simulink model "inverted_pendulum"  (R2021a)
settings: Solver=VariableStepAuto  StartTime=0.0  StopTime=5  FixedStep=0.001  MaxStep=0.0001  RelTol=1e-3
values from neighbouring files (symbols this model uses):
  A = [0          1       0       0 ... (first row only)    [Data.m]
  B = [0 0 0 1/La]'    [Data.m]
  beta = g*(mp*L1 + mw * L2)    (= 0.64746)    [Data.m]    (also in uncertainty.m = g*(mp*L1 + mw * L2))
  bm = 0.018    [Data.m]    (also in uncertainty.m = ureal('bm', 0.018, 'percent', 20))
  bp = 0.038    [Data.m]    (also in uncertainty.m = ureal('bp', 0.038, 'percent', 100))
  C = [1 0 0 0]    [Data.m]
  fs_IMU = 1000    [Data.m]
  g = 9.81    [Data.m]    (also in uncertainty.m)
  ideal_acc_height = 0    [Data.m]
  J1 = Jw + Jp_O    (= 0.0170488)    [Data.m]    (also in uncertainty.m = Jw + Jp_O)
  Jw = J_motor + J_wheel    (= 0.0042488)    [Data.m]    (also in uncertainty.m = J_motor + J_wheel)
  Ke = 1.66e-2    (= 0.0166)    [Data.m]    (also in gear_test.m = gear*Kt; uncertainty.m = ureal('Ke', 1.66e-2, 'percent', 20))
  Ksw = 0.035    [Data.m]    (also in Ksw_test.m = Ksw_v(i))
  Kt = 1    [Data.m]    (also in gear_test.m = gear*0.876; uncertainty.m = ureal('Kt', 1, 'percent', 20))
  L = L_t'    [Data.m]
  La = 3.2e-3    (= 0.0032)    [Data.m]    (also in uncertainty.m = ureal('La', 3.2e-3, 'percent', 20))
  Ra = 40.8    [Data.m]    (also in uncertainty.m = ureal('Ra', 40.8, 'percent', 20))
  real_acc_height = 0.02    [Data.m]
  V_nom = 24    [Data.m]    (also in uncertainty.m)
  wd_IMU = 30000*2*pi    (= 188495.559215)    [Data.m]
  wn = sqrt(mp*g*L2/Jp_O)    [Data.m]
  x0 = [0.3 0 0 0]    [Data.m]
  x0_sw = [pi 0 0 0]    [Data.m]    (also in phase_space.m = [-pi 0 0 0])
undefined symbols (not defined in the file or in its folder): acc_bias, gyro_bias, K
libraries: spsFirstOrderFilterLib x18, simulink x9, dspsigops x2
(part 2 of 2)

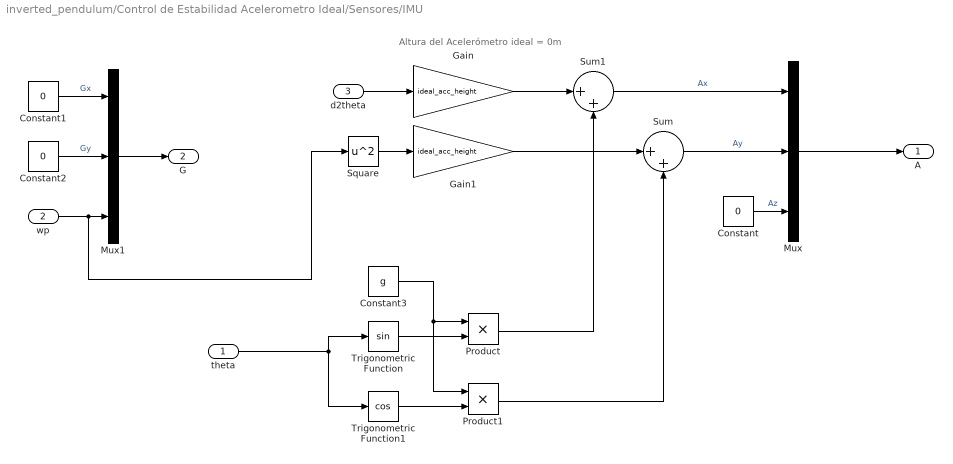
== system inverted_pendulum/Control de Estabilidad Acelerometro Ideal/Sensores/IMU ==
  note: Altura del Acelerómetro ideal = 0m
  theta : Inport
  wp : Inport  Port=2
  d2theta : Inport  Port=3
  Constant : Constant  Value=0
  Constant1 : Constant  Value=0
  Constant2 : Constant  Value=0
  Constant3 : Constant  Value=g
  Gain : Gain  Gain=ideal_acc_height
  Gain1 : Gain  Gain=ideal_acc_height
  Mux : Mux  Inputs=3
  Mux1 : Mux  Inputs=3
  Product : Product
  Product1 : Product
  Square : Math  Operator=square  SaturateOnIntegerOverflow=on
  Sum : Sum  Inputs=|++
  Sum1 : Sum  Inputs=|++
  Trigonometric Function : Trigonometry
  Trigonometric Function1 : Trigonometry  Operator=cos
  A : Outport
  G : Outport  Port=2
  wires:
  Mux/1 -> A/1
  Mux1/1 -> G/1
  Sum/1 -> Mux/2  "Ay"
  Constant/1 -> Mux/3  "Az"
  Sum1/1 -> Mux/1  "Ax"
  Constant2/1 -> Mux1/2  "Gy"
  Constant1/1 -> Mux1/1  "Gx"
  wp/1 -> Square/1, Mux1/3
  Trigonometric Function/1 -> Product/2
  Trigonometric Function1/1 -> Product1/2
  Constant3/1 -> Product1/1, Product/1
  Product1/1 -> Sum/2
  Product/1 -> Sum1/2
  Gain1/1 -> Sum/1
  theta/1 -> Trigonometric Function1/1, Trigonometric Function/1
  Gain/1 -> Sum1/1
  d2theta/1 -> Gain/1
  Square/1 -> Gain1/1

== system inverted_pendulum/Control de Estabilidad Acelerometro Real/Péndulo invertido NL/Motor CC + Rueda ==
  note: Rueda
  note: Motor CC
  V : Inport
  Gain : Gain  Gain=1/Jw
  Gain1 : Gain  Gain=bm
  Gain2 : Gain  Gain=Kt
  Gain3 : Gain  Gain=1/La
  Gain4 : Gain  Gain=Ra
  Gain5 : Gain  Gain=Ke
  Integrator ia : Integrator  InitialCondition=x0(4)
  Integrator wm : Integrator  InitialCondition=x0(3)
  Sum : Sum  Inputs=|+-
  Sum1 : Sum  Inputs=|+--
  wm : Outport
  ia : Outport  Port=2
  wires:
  Sum/1 -> Gain/1
  Gain/1 -> Integrator wm/1  "d2phi"
  Integrator wm/1 -> wm/1, Gain1/1, Gain5/1  "wm"
  Gain1/1 -> Sum/2
  Gain2/1 -> Sum/1
  Integrator ia/1 -> ia/1, Gain4/1, Gain2/1  "ia"
  Gain3/1 -> Integrator ia/1  "di/dt"
  Sum1/1 -> Gain3/1
  Gain4/1 -> Sum1/3
  V/1 -> Sum1/1  "V"
  Gain5/1 -> Sum1/2

== system inverted_pendulum/Control de Estabilidad Acelerometro Real/Péndulo invertido NL/Péndulo invertido ==
  note: Péndulo
  note: Fricción del motor
  note: Torque del motor
  wm : Inport
  ia : Inport  Port=2
  Gain : Gain  Gain=1/J1
  Gain1 : Gain  Gain=beta
  Gain2 : Gain  Gain=Kt
  Gain3 : Gain  Gain=bp
  Gain4 : Gain  Gain=bm
  Integrator Theta : Integrator  InitialCondition=x0(1)  WrappedStateUpperValue=2*pi  WrappedStateLowerValue=0
  Integrator wp : Integrator  InitialCondition=x0(2)
  Sum : Sum  Inputs=+-+-
  Trigonometric Function1 : Trigonometry
  theta : Outport
  wp : Outport  Port=2
  d2theta : Outport  Port=3
  wires:
  Trigonometric Function1/1 -> Gain1/1
  Gain/1 -> d2theta/1, Integrator wp/1  "d2theta"
  Sum/1 -> Gain/1
  Integrator Theta/1 -> Trigonometric Function1/1, theta/1  "theta"
  Integrator wp/1 -> wp/1, Gain3/1, Integrator Theta/1  "wp"
  Gain3/1 -> Sum/4
  Gain1/1 -> Sum/3
  ia/1 -> Gain2/1
  Gain2/1 -> Sum/2
  wm/1 -> Gain4/1
  Gain4/1 -> Sum/1

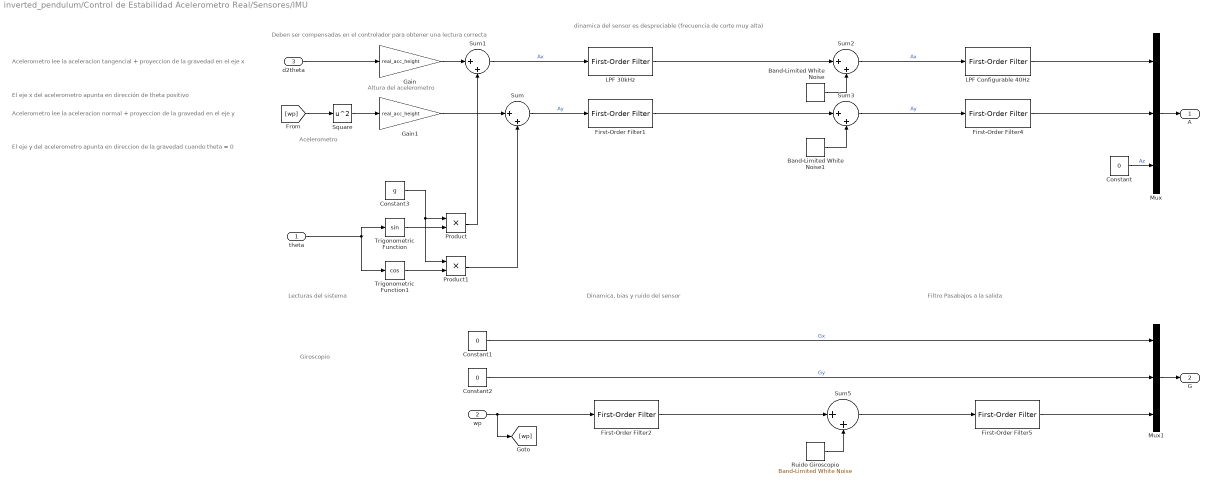
== system inverted_pendulum/Control de Estabilidad Acelerometro Real/Sensores/IMU ==
  note: dinamica del sensor es despreciable (frecuencia de corte muy alta)
  note: Dinamica, bias y ruido del sensor
  note: Lecturas del sistema
  note: Acelerometro
  note: Deben ser compensadas en el controlador para obtener una lectura correcta
  note: Acelerometro lee la aceleracion tangencial + proyeccion de la gravedad en el eje x
  note: Altura del acelerometro
  note: El eje y del acelerometro apunta en direccion de la gravedad cuando theta = 0
  note: El eje x del acelerometro apunta en dirección de theta positivo
  note: Acelerometro lee la aceleracion normal + proyeccion de la gravedad en el eje y
  note: Giroscopio
  note: Filtro Pasabajos a la salida
  theta : Inport
  wp : Inport  Port=2
  d2theta : Inport  Port=3
  Band-Limited White Noise : simulink/Sources/Band-Limited White Noise  Cov=acc_noise_power  Ts=1/fs_IMU  seed=[23341]
  Band-Limited White Noise1 : simulink/Sources/Band-Limited White Noise  Cov=acc_noise_power  Ts=1/fs_IMU  seed=[23341]
  Constant : Constant  Value=0
  Constant1 : Constant  Value=0
  Constant2 : Constant  Value=0
  Constant3 : Constant  Value=g
  First-Order Filter{1..2,4..5} (4 alike) : spsFirstOrderFilterLib/First-Order Filter  FilterType=Lowpass  Tc=2*pi/wd_IMU  Ts=0  Initialize=on  Vac_Init=[0, 0, 60]  Vdc_Init=0  PlotResponse=off  FreqRange="[0,  200,  1]"
  Gain : Gain  Gain=real_acc_height
  Gain1 : Gain  Gain=real_acc_height
  LPF 30kHz : spsFirstOrderFilterLib/First-Order Filter  FilterType=Lowpass  Tc=2*pi/wd_IMU  Ts=0  Initialize=on  Vac_Init=[0, 0, 60]  Vdc_Init=0  PlotResponse=off  FreqRange="[0,  200,  1]"
  LPF Configurable 40Hz : spsFirstOrderFilterLib/First-Order Filter  FilterType=Lowpass  Tc=2*pi/wd_IMU  Ts=0  Initialize=on  Vac_Init=[0, 0, 60]  Vdc_Init=0  PlotResponse=off  FreqRange="[0,  200,  1]"
  Mux : Mux  Inputs=3
  Mux1 : Mux  Inputs=3
  Product : Product
  Product1 : Product
  Ruido Giroscopio : simulink/Sources/Band-Limited White Noise  Cov=gyro_noise_power  Ts=1/fs_IMU  seed=[23341]
  Square : Math  Operator=square  SaturateOnIntegerOverflow=on
  Sum{,1..3,5} (5 alike) : Sum  Inputs=|++
  Trigonometric Function : Trigonometry
  Trigonometric Function1 : Trigonometry  Operator=cos
  A : Outport
  G : Outport  Port=2
  wires:
  Constant2/1 -> Mux1/2  "Gy"
  Constant1/1 -> Mux1/1  "Gx"
  Trigonometric Function/1 -> Product/2
  Trigonometric Function1/1 -> Product1/2
  Constant3/1 -> Product1/1, Product/1
  Product1/1 -> Sum/2
  Product/1 -> Sum1/2
  Gain1/1 -> Sum/1
  theta/1 -> Trigonometric Function1/1, Trigonometric Function/1
  Gain/1 -> Sum1/1
  d2theta/1 -> Gain/1
  Square/1 -> Gain1/1
  Constant/1 -> Mux/3  "Az"
  Sum1/1 -> LPF 30kHz/1  "Ax"
  Band-Limited White Noise/1 -> Sum2/2
  Band-Limited White Noise1/1 -> Sum3/2
  Ruido Giroscopio/1 -> Sum5/2
  First-Order Filter1/1 -> Sum3/1
  First-Order Filter2/1 -> Sum5/1
  wp/1 -> First-Order Filter2/1, [wp]
  Mux/1 -> A/1
  Mux1/1 -> G/1
  Sum5/1 -> First-Order Filter5/1
  Sum2/1 -> LPF Configurable 40Hz/1  "Ax"
  Sum3/1 -> First-Order Filter4/1  "Ay"
  [wp] -> Square/1
  Sum/1 -> First-Order Filter1/1  "Ay"
  LPF 30kHz/1 -> Sum2/1
  First-Order Filter4/1 -> Mux/2
  LPF Configurable 40Hz/1 -> Mux/1
  First-Order Filter5/1 -> Mux1/3

== system inverted_pendulum/Control de Estabilidad Sensores ideales/Péndulo invertido NL/Motor CC + Rueda ==
  note: Rueda
  note: Motor CC
  V : Inport
  Gain : Gain  Gain=1/Jw
  Gain1 : Gain  Gain=bm
  Gain2 : Gain  Gain=Kt
  Gain3 : Gain  Gain=1/La
  Gain4 : Gain  Gain=Ra
  Gain5 : Gain  Gain=Ke
  Integrator ia : Integrator  InitialCondition=x0(4)
  Integrator wm : Integrator  InitialCondition=x0(3)
  Sum : Sum  Inputs=|+-
  Sum1 : Sum  Inputs=|+--
  wm : Outport
  ia : Outport  Port=2
  wires:
  Sum/1 -> Gain/1
  Gain/1 -> Integrator wm/1  "d2phi"
  Integrator wm/1 -> wm/1, Gain1/1, Gain5/1  "wm"
  Gain1/1 -> Sum/2
  Gain2/1 -> Sum/1
  Integrator ia/1 -> ia/1, Gain4/1, Gain2/1  "ia"
  Gain3/1 -> Integrator ia/1  "di/dt"
  Sum1/1 -> Gain3/1
  Gain4/1 -> Sum1/3
  V/1 -> Sum1/1  "V"
  Gain5/1 -> Sum1/2

== system inverted_pendulum/Control de Estabilidad Sensores ideales/Péndulo invertido NL/Péndulo invertido ==
  note: Péndulo
  note: Fricción del motor
  note: Torque del motor
  wm : Inport
  ia : Inport  Port=2
  Gain : Gain  Gain=1/J1
  Gain1 : Gain  Gain=beta
  Gain2 : Gain  Gain=Kt
  Gain3 : Gain  Gain=bp
  Gain4 : Gain  Gain=bm
  Integrator Theta : Integrator  InitialCondition=x0(1)  WrappedStateUpperValue=2*pi  WrappedStateLowerValue=0
  Integrator wp : Integrator  InitialCondition=x0(2)
  Sum : Sum  Inputs=+-+-
  Trigonometric Function1 : Trigonometry
  theta : Outport
  wp : Outport  Port=2
  d2theta : Outport  Port=3
  wires:
  Trigonometric Function1/1 -> Gain1/1
  Gain/1 -> d2theta/1, Integrator wp/1  "d2theta"
  Sum/1 -> Gain/1
  Integrator Theta/1 -> Trigonometric Function1/1, theta/1  "theta"
  Integrator wp/1 -> wp/1, Gain3/1, Integrator Theta/1  "wp"
  Gain3/1 -> Sum/4
  Gain1/1 -> Sum/3
  ia/1 -> Gain2/1
  Gain2/1 -> Sum/2
  wm/1 -> Gain4/1
  Gain4/1 -> Sum/1

== system inverted_pendulum/Control Híbrido Acelerómetro Real/Control Híbrido/Balanceo/Cálculo de Energía ==
  note: Energía Potencial
  note: Energía Cinética
  note: Energía instantánea
  note: Energía en theta = 0
  theta : Inport
  wp : Inport  Port=2
  Constant : Constant
  Constant1 : Constant  Value=wn^2
  Constant2 : Constant  Value=2
  Divide : Product  Inputs=*/
  Gain : Gain  Gain=1/2
  Square : Math  Operator=square  SaturateOnIntegerOverflow=on
  Sum : Sum  Inputs=|+-
  Sum1 : Sum  Inputs=+++
  Trigonometric Function : Trigonometry  Operator=cos
  Eref-E : Outport
  wires:
  Sum/1 -> Eref-E/1
  Constant2/1 -> Sum/1  "Eref"
  Sum1/1 -> Sum/2  "E"
  Constant/1 -> Sum1/3
  Trigonometric Function/1 -> Sum1/2
  theta/1 -> Trigonometric Function/1  "theta"
  Divide/1 -> Square/1
  wp/1 -> Divide/1  "wp"
  Constant1/1 -> Divide/2  "wn"
  Square/1 -> Gain/1
  Gain/1 -> Sum1/1

== system inverted_pendulum/Control Híbrido Sensores Ideales/Control Híbrido/Balanceo/Cálculo de Energía ==
  note: Energía Potencial
  note: Energía Cinética
  note: Energía instantánea
  note: Energía en theta = 0
  theta : Inport
  wp : Inport  Port=2
  Constant : Constant
  Constant1 : Constant  Value=wn
  Constant2 : Constant  Value=2
  Divide : Product  Inputs=*/
  Gain : Gain  Gain=1/2
  Product : Product
  Sum : Sum  Inputs=|+-
  Sum1 : Sum  Inputs=+++
  Trigonometric Function : Trigonometry  Operator=cos
  Eref-E : Outport
  wires:
  Sum/1 -> Eref-E/1
  Constant2/1 -> Sum/1  "Eref"
  Sum1/1 -> Sum/2  "E"
  Constant/1 -> Sum1/3
  Trigonometric Function/1 -> Sum1/2
  theta/1 -> Trigonometric Function/1  "theta"
  Divide/1 -> Product/1, Product/2
  wp/1 -> Divide/1  "wp"
  Constant1/1 -> Divide/2  "wn"
  Product/1 -> Gain/1
  Gain/1 -> Sum1/1

== matlab function inverted_pendulum/Control de Estabilidad Acelerometro Real/Acondicionamiento de Señal/MATLAB Function ==
  data: theta_acc input; theta_filtered output; Gz input; theta_last input
function theta_filtered = complementaryFilter(theta_acc, Gz, theta_last)
alpha = 0.9;
theta_gy = Gz * 0.0001;
theta_filtered = theta_acc*(1-alpha) + alpha * (theta_last + theta_gy);

%%%%FILTOR PASAALTO Y PASA BAJO

== matlab function inverted_pendulum/Control de Balanceo Acelerometro Real/Acondicionamiento de Señal/MATLAB Function ==
  data: theta_acc input; theta_filtered output; Gz input; theta_last input
function theta_filtered = complementaryFilter(theta_acc, Gz, theta_last)
alpha = 0.9;
theta_gy = Gz * 0.0001;
theta_filtered = theta_acc*(1-alpha) + alpha * (theta_last + theta_gy);

== matlab function inverted_pendulum/Control de Estabilidad Acelerometro Real/Estimación de estados/MATLAB Function ==
  data: x input; F output; A input
function F = CampoVectorial(x, A)

k = A(2,1);
A(2,1) = 0;
F = A*x;

F(2) = F(2) + k * sin(x(1));

== matlab function inverted_pendulum/Control de Estabilidad Acelerometro Ideal/Estimación de estados/MATLAB Function ==
  data: x input; F output; A input
function F = CampoVectorial(x, A)

k = A(2,1);
A(2,1) = 0;
F = A*x;

F(2) = F(2) + k * sin(x(1));

== matlab function inverted_pendulum/Control Híbrido Acelerómetro Real/Acondicionamiento de Señal/MATLAB Function ==
  data: theta_acc input; theta_filtered output; Gz input; theta_last input
function theta_filtered = complementaryFilter(theta_acc, Gz, theta_last)
alpha = 0.9;
theta_gy = Gz * 0.0001;
theta_filtered = theta_acc*(1-alpha) + alpha * (theta_last + theta_gy);

== matlab function inverted_pendulum/Control Híbrido Acelerómetro Real/Estimación de estados/MATLAB Function ==
  data: x input; F output; A input
function F = CampoVectorial(x, A)

k = A(2,1);
A(2,1) = 0;
F = A*x;

F(2) = F(2) + k * sin(x(1));

== matlab function inverted_pendulum/Control de Balanceo Acelerometro Real/Estimación de estados/MATLAB Function ==
  data: x input; F output; A input
function F = CampoVectorial(x, A)

k = A(2,1);
A(2,1) = 0;
F = A*x;

F(2) = F(2) + k * sin(x(1));
